simulink model "REGISTROS_64_BITS_02"  (R2022a)
settings: Solver=VariableStepAuto  StartTime=0.0  StopTime=10.0  RelTol=1e-3
undefined symbols (not defined in the file or in its folder): xc7z010iclg225
libraries: hdlBasic x6609, vmcUtilities x1
(part 20 of 23)

== system REGISTROS_64_BITS_02/REGISTRO_64_BITS_2/Q_OUT_32_BIT1 ==
  Q_OUT_0 (1 BIT) : Inport
  Q_OUT_1 (1 BIT) : Inport  Port=2
  Q_OUT_2 (1 BIT) : Inport  Port=3
  Q_OUT_3 (1 BIT) : Inport  Port=4
  Q_OUT_4 (1 BIT) : Inport  Port=5
  Q_OUT_5 (1 BIT) : Inport  Port=6
  Q_OUT_6 (1 BIT) : Inport  Port=7
  Q_OUT_7 (1 BIT) : Inport  Port=8
  Q_OUT_8 (1 BIT) : Inport  Port=9
  Q_OUT_9 (1 BIT) : Inport  Port=10
  Q_OUT_10 (1 BIT) : Inport  Port=11
  Q_OUT_11 (1 BIT) : Inport  Port=12
  Q_OUT_12 (1 BIT) : Inport  Port=13
  Q_OUT_13 (1 BIT) : Inport  Port=14
  Q_OUT_14 (1 BIT) : Inport  Port=15
  Q_OUT_15 (1 BIT) : Inport  Port=16
  Q_OUT_16 (1 BIT) : Inport  Port=17
  Q_OUT_17 (1 BIT) : Inport  Port=18
  Q_OUT_18 (1 BIT) : Inport  Port=19
  Q_OUT_19 (1 BIT) : Inport  Port=20
  Q_OUT_20 (1 BIT) : Inport  Port=21
  Q_OUT_21 (1 BIT) : Inport  Port=22
  Q_OUT_22 (1 BIT) : Inport  Port=23
  Q_OUT_23 (1 BIT) : Inport  Port=24
  Q_OUT_24 (1 BIT) : Inport  Port=25
  Q_OUT_25 (1 BIT) : Inport  Port=26
  Q_OUT_26 (1 BIT) : Inport  Port=27
  Q_OUT_27 (1 BIT) : Inport  Port=28
  Q_OUT_28 (1 BIT) : Inport  Port=29
  Q_OUT_29 (1 BIT) : Inport  Port=30
  Q_OUT_30 (1 BIT) : Inport  Port=31
  Q_OUT_31 (1 BIT) : Inport  Port=32
  Concat{1,3,6,8..30} (26 alike) : hdlBasic/Concat  num_inputs=2  XmcBlockStatus=1  maskContainerNames=group1  block_type=concat  block_config=sysgen:Concat_config
  IN_00 : hdlBasic/Concat  num_inputs=2  XmcBlockStatus=1  maskContainerNames=group1  block_type=concat  block_config=sysgen:Concat_config
  IN_01 : hdlBasic/Concat  num_inputs=2  XmcBlockStatus=1  maskContainerNames=group1  block_type=concat  block_config=sysgen:Concat_config
  IN_02 : hdlBasic/Concat  num_inputs=2  XmcBlockStatus=1  maskContainerNames=group1  block_type=concat  block_config=sysgen:Concat_config
  IN_03 : hdlBasic/Concat  num_inputs=2  XmcBlockStatus=1  maskContainerNames=group1  block_type=concat  block_config=sysgen:Concat_config
  IN_04 : hdlBasic/Concat  num_inputs=2  XmcBlockStatus=1  maskContainerNames=group1  block_type=concat  block_config=sysgen:Concat_config
  Q (32 BIT) : Outport
  wires:
  IN_01/1 -> Concat3/2
  Concat10/1 -> Concat12/1
  Concat27/1 -> Concat20/2
  Concat19/1 -> Concat21/2
  Concat22/1 -> Concat1/2
  Concat28/1 -> Concat30/1
  Concat11/1 -> Concat12/2
  Concat29/1 -> Concat30/2
  Concat21/1 -> Concat22/2
  IN_00/1 -> Concat3/1
  Concat3/1 -> Concat13/1
  Concat20/1 -> Concat22/1
  Concat17/1 -> Concat19/1
  Concat26/1 -> Concat27/2
  Concat6/1 -> Concat13/2
  Concat13/1 -> Concat15/1
  Concat30/1 -> Concat21/1
  Concat24/1 -> Concat20/1
  Concat16/1 -> Concat24/1
  Concat23/1 -> Concat24/2
  Concat18/1 -> Concat19/2
  Concat25/1 -> Concat27/1
  IN_02/1 -> Concat6/1
  IN_03/1 -> Concat6/2
  Concat9/1 -> Concat14/1
  Concat15/1 -> Concat1/1
  Concat8/1 -> Concat9/2
  IN_04/1 -> Concat9/1
  Concat14/1 -> Concat15/2
  Concat12/1 -> Concat14/2
  Concat1/1 -> Q (32 BIT)/1
  Q_OUT_31 (1 BIT)/1 -> IN_00/1
  Q_OUT_30 (1 BIT)/1 -> IN_00/2
  Q_OUT_29 (1 BIT)/1 -> IN_01/1
  Q_OUT_28 (1 BIT)/1 -> IN_01/2
  Q_OUT_27 (1 BIT)/1 -> IN_02/1
  Q_OUT_26 (1 BIT)/1 -> IN_02/2
  Q_OUT_25 (1 BIT)/1 -> IN_03/1
  Q_OUT_24 (1 BIT)/1 -> IN_03/2
  Q_OUT_23 (1 BIT)/1 -> IN_04/1
  Q_OUT_22 (1 BIT)/1 -> IN_04/2
  Q_OUT_21 (1 BIT)/1 -> Concat8/1
  Q_OUT_20 (1 BIT)/1 -> Concat8/2
  Q_OUT_19 (1 BIT)/1 -> Concat10/1
  Q_OUT_18 (1 BIT)/1 -> Concat10/2
  Q_OUT_17 (1 BIT)/1 -> Concat11/1
  Q_OUT_16 (1 BIT)/1 -> Concat11/2
  Q_OUT_15 (1 BIT)/1 -> Concat16/1
  Q_OUT_14 (1 BIT)/1 -> Concat16/2
  Q_OUT_13 (1 BIT)/1 -> Concat23/1
  Q_OUT_12 (1 BIT)/1 -> Concat23/2
  Q_OUT_11 (1 BIT)/1 -> Concat25/1
  Q_OUT_10 (1 BIT)/1 -> Concat25/2
  Q_OUT_9 (1 BIT)/1 -> Concat26/1
  Q_OUT_8 (1 BIT)/1 -> Concat26/2
  Q_OUT_7 (1 BIT)/1 -> Concat28/1
  Q_OUT_6 (1 BIT)/1 -> Concat28/2
  Q_OUT_5 (1 BIT)/1 -> Concat29/1
  Q_OUT_4 (1 BIT)/1 -> Concat29/2
  Q_OUT_3 (1 BIT)/1 -> Concat17/1
  Q_OUT_2 (1 BIT)/1 -> Concat17/2
  Q_OUT_1 (1 BIT)/1 -> Concat18/1
  Q_OUT_0 (1 BIT)/1 -> Concat18/2

== system REGISTROS_64_BITS_02/REGISTRO_64_BITS_2/Q_OUT_32_BIT2 ==
  Q_OUT_0 (1 BIT) : Inport
  Q_OUT_1 (1 BIT) : Inport  Port=2
  Q_OUT_2 (1 BIT) : Inport  Port=3
  Q_OUT_3 (1 BIT) : Inport  Port=4
  Q_OUT_4 (1 BIT) : Inport  Port=5
  Q_OUT_5 (1 BIT) : Inport  Port=6
  Q_OUT_6 (1 BIT) : Inport  Port=7
  Q_OUT_7 (1 BIT) : Inport  Port=8
  Q_OUT_8 (1 BIT) : Inport  Port=9
  Q_OUT_9 (1 BIT) : Inport  Port=10
  Q_OUT_10 (1 BIT) : Inport  Port=11
  Q_OUT_11 (1 BIT) : Inport  Port=12
  Q_OUT_12 (1 BIT) : Inport  Port=13
  Q_OUT_13 (1 BIT) : Inport  Port=14
  Q_OUT_14 (1 BIT) : Inport  Port=15
  Q_OUT_15 (1 BIT) : Inport  Port=16
  Q_OUT_16 (1 BIT) : Inport  Port=17
  Q_OUT_17 (1 BIT) : Inport  Port=18
  Q_OUT_18 (1 BIT) : Inport  Port=19
  Q_OUT_19 (1 BIT) : Inport  Port=20
  Q_OUT_20 (1 BIT) : Inport  Port=21
  Q_OUT_21 (1 BIT) : Inport  Port=22
  Q_OUT_22 (1 BIT) : Inport  Port=23
  Q_OUT_23 (1 BIT) : Inport  Port=24
  Q_OUT_24 (1 BIT) : Inport  Port=25
  Q_OUT_25 (1 BIT) : Inport  Port=26
  Q_OUT_26 (1 BIT) : Inport  Port=27
  Q_OUT_27 (1 BIT) : Inport  Port=28
  Q_OUT_28 (1 BIT) : Inport  Port=29
  Q_OUT_29 (1 BIT) : Inport  Port=30
  Q_OUT_30 (1 BIT) : Inport  Port=31
  Q_OUT_31 (1 BIT) : Inport  Port=32
  Concat{1,3,6,8..30} (26 alike) : hdlBasic/Concat  num_inputs=2  XmcBlockStatus=1  maskContainerNames=group1  block_type=concat  block_config=sysgen:Concat_config
  IN_00 : hdlBasic/Concat  num_inputs=2  XmcBlockStatus=1  maskContainerNames=group1  block_type=concat  block_config=sysgen:Concat_config
  IN_01 : hdlBasic/Concat  num_inputs=2  XmcBlockStatus=1  maskContainerNames=group1  block_type=concat  block_config=sysgen:Concat_config
  IN_02 : hdlBasic/Concat  num_inputs=2  XmcBlockStatus=1  maskContainerNames=group1  block_type=concat  block_config=sysgen:Concat_config
  IN_03 : hdlBasic/Concat  num_inputs=2  XmcBlockStatus=1  maskContainerNames=group1  block_type=concat  block_config=sysgen:Concat_config
  IN_04 : hdlBasic/Concat  num_inputs=2  XmcBlockStatus=1  maskContainerNames=group1  block_type=concat  block_config=sysgen:Concat_config
  Q (32 BIT) : Outport
  wires:
  IN_01/1 -> Concat3/2
  Concat10/1 -> Concat12/1
  Concat27/1 -> Concat20/2
  Concat19/1 -> Concat21/2
  Concat22/1 -> Concat1/2
  Concat28/1 -> Concat30/1
  Concat11/1 -> Concat12/2
  Concat29/1 -> Concat30/2
  Concat21/1 -> Concat22/2
  IN_00/1 -> Concat3/1
  Concat3/1 -> Concat13/1
  Concat20/1 -> Concat22/1
  Concat17/1 -> Concat19/1
  Concat26/1 -> Concat27/2
  Concat6/1 -> Concat13/2
  Concat13/1 -> Concat15/1
  Concat30/1 -> Concat21/1
  Concat24/1 -> Concat20/1
  Concat16/1 -> Concat24/1
  Concat23/1 -> Concat24/2
  Concat18/1 -> Concat19/2
  Concat25/1 -> Concat27/1
  IN_02/1 -> Concat6/1
  IN_03/1 -> Concat6/2
  Concat9/1 -> Concat14/1
  Concat15/1 -> Concat1/1
  Concat8/1 -> Concat9/2
  IN_04/1 -> Concat9/1
  Concat14/1 -> Concat15/2
  Concat12/1 -> Concat14/2
  Concat1/1 -> Q (32 BIT)/1
  Q_OUT_31 (1 BIT)/1 -> IN_00/1
  Q_OUT_30 (1 BIT)/1 -> IN_00/2
  Q_OUT_29 (1 BIT)/1 -> IN_01/1
  Q_OUT_28 (1 BIT)/1 -> IN_01/2
  Q_OUT_27 (1 BIT)/1 -> IN_02/1
  Q_OUT_26 (1 BIT)/1 -> IN_02/2
  Q_OUT_25 (1 BIT)/1 -> IN_03/1
  Q_OUT_24 (1 BIT)/1 -> IN_03/2
  Q_OUT_23 (1 BIT)/1 -> IN_04/1
  Q_OUT_22 (1 BIT)/1 -> IN_04/2
  Q_OUT_21 (1 BIT)/1 -> Concat8/1
  Q_OUT_20 (1 BIT)/1 -> Concat8/2
  Q_OUT_19 (1 BIT)/1 -> Concat10/1
  Q_OUT_18 (1 BIT)/1 -> Concat10/2
  Q_OUT_17 (1 BIT)/1 -> Concat11/1
  Q_OUT_16 (1 BIT)/1 -> Concat11/2
  Q_OUT_15 (1 BIT)/1 -> Concat16/1
  Q_OUT_14 (1 BIT)/1 -> Concat16/2
  Q_OUT_13 (1 BIT)/1 -> Concat23/1
  Q_OUT_12 (1 BIT)/1 -> Concat23/2
  Q_OUT_11 (1 BIT)/1 -> Concat25/1
  Q_OUT_10 (1 BIT)/1 -> Concat25/2
  Q_OUT_9 (1 BIT)/1 -> Concat26/1
  Q_OUT_8 (1 BIT)/1 -> Concat26/2
  Q_OUT_7 (1 BIT)/1 -> Concat28/1
  Q_OUT_6 (1 BIT)/1 -> Concat28/2
  Q_OUT_5 (1 BIT)/1 -> Concat29/1
  Q_OUT_4 (1 BIT)/1 -> Concat29/2
  Q_OUT_3 (1 BIT)/1 -> Concat17/1
  Q_OUT_2 (1 BIT)/1 -> Concat17/2
  Q_OUT_1 (1 BIT)/1 -> Concat18/1
  Q_OUT_0 (1 BIT)/1 -> Concat18/2

== system REGISTROS_64_BITS_02/REGISTRO_64_BITS_20/Q_OUT_32_BIT1 ==
  Q_OUT_0 (1 BIT) : Inport
  Q_OUT_1 (1 BIT) : Inport  Port=2
  Q_OUT_2 (1 BIT) : Inport  Port=3
  Q_OUT_3 (1 BIT) : Inport  Port=4
  Q_OUT_4 (1 BIT) : Inport  Port=5
  Q_OUT_5 (1 BIT) : Inport  Port=6
  Q_OUT_6 (1 BIT) : Inport  Port=7
  Q_OUT_7 (1 BIT) : Inport  Port=8
  Q_OUT_8 (1 BIT) : Inport  Port=9
  Q_OUT_9 (1 BIT) : Inport  Port=10
  Q_OUT_10 (1 BIT) : Inport  Port=11
  Q_OUT_11 (1 BIT) : Inport  Port=12
  Q_OUT_12 (1 BIT) : Inport  Port=13
  Q_OUT_13 (1 BIT) : Inport  Port=14
  Q_OUT_14 (1 BIT) : Inport  Port=15
  Q_OUT_15 (1 BIT) : Inport  Port=16
  Q_OUT_16 (1 BIT) : Inport  Port=17
  Q_OUT_17 (1 BIT) : Inport  Port=18
  Q_OUT_18 (1 BIT) : Inport  Port=19
  Q_OUT_19 (1 BIT) : Inport  Port=20
  Q_OUT_20 (1 BIT) : Inport  Port=21
  Q_OUT_21 (1 BIT) : Inport  Port=22
  Q_OUT_22 (1 BIT) : Inport  Port=23
  Q_OUT_23 (1 BIT) : Inport  Port=24
  Q_OUT_24 (1 BIT) : Inport  Port=25
  Q_OUT_25 (1 BIT) : Inport  Port=26
  Q_OUT_26 (1 BIT) : Inport  Port=27
  Q_OUT_27 (1 BIT) : Inport  Port=28
  Q_OUT_28 (1 BIT) : Inport  Port=29
  Q_OUT_29 (1 BIT) : Inport  Port=30
  Q_OUT_30 (1 BIT) : Inport  Port=31
  Q_OUT_31 (1 BIT) : Inport  Port=32
  Concat{1,3,6,8..30} (26 alike) : hdlBasic/Concat  num_inputs=2  XmcBlockStatus=1  maskContainerNames=group1  block_type=concat  block_config=sysgen:Concat_config
  IN_00 : hdlBasic/Concat  num_inputs=2  XmcBlockStatus=1  maskContainerNames=group1  block_type=concat  block_config=sysgen:Concat_config
  IN_01 : hdlBasic/Concat  num_inputs=2  XmcBlockStatus=1  maskContainerNames=group1  block_type=concat  block_config=sysgen:Concat_config
  IN_02 : hdlBasic/Concat  num_inputs=2  XmcBlockStatus=1  maskContainerNames=group1  block_type=concat  block_config=sysgen:Concat_config
  IN_03 : hdlBasic/Concat  num_inputs=2  XmcBlockStatus=1  maskContainerNames=group1  block_type=concat  block_config=sysgen:Concat_config
  IN_04 : hdlBasic/Concat  num_inputs=2  XmcBlockStatus=1  maskContainerNames=group1  block_type=concat  block_config=sysgen:Concat_config
  Q (32 BIT) : Outport
  wires:
  IN_01/1 -> Concat3/2
  Concat10/1 -> Concat12/1
  Concat27/1 -> Concat20/2
  Concat19/1 -> Concat21/2
  Concat22/1 -> Concat1/2
  Concat28/1 -> Concat30/1
  Concat11/1 -> Concat12/2
  Concat29/1 -> Concat30/2
  Concat21/1 -> Concat22/2
  IN_00/1 -> Concat3/1
  Concat3/1 -> Concat13/1
  Concat20/1 -> Concat22/1
  Concat17/1 -> Concat19/1
  Concat26/1 -> Concat27/2
  Concat6/1 -> Concat13/2
  Concat13/1 -> Concat15/1
  Concat30/1 -> Concat21/1
  Concat24/1 -> Concat20/1
  Concat16/1 -> Concat24/1
  Concat23/1 -> Concat24/2
  Concat18/1 -> Concat19/2
  Concat25/1 -> Concat27/1
  IN_02/1 -> Concat6/1
  IN_03/1 -> Concat6/2
  Concat9/1 -> Concat14/1
  Concat15/1 -> Concat1/1
  Concat8/1 -> Concat9/2
  IN_04/1 -> Concat9/1
  Concat14/1 -> Concat15/2
  Concat12/1 -> Concat14/2
  Concat1/1 -> Q (32 BIT)/1
  Q_OUT_31 (1 BIT)/1 -> IN_00/1
  Q_OUT_30 (1 BIT)/1 -> IN_00/2
  Q_OUT_29 (1 BIT)/1 -> IN_01/1
  Q_OUT_28 (1 BIT)/1 -> IN_01/2
  Q_OUT_27 (1 BIT)/1 -> IN_02/1
  Q_OUT_26 (1 BIT)/1 -> IN_02/2
  Q_OUT_25 (1 BIT)/1 -> IN_03/1
  Q_OUT_24 (1 BIT)/1 -> IN_03/2
  Q_OUT_23 (1 BIT)/1 -> IN_04/1
  Q_OUT_22 (1 BIT)/1 -> IN_04/2
  Q_OUT_21 (1 BIT)/1 -> Concat8/1
  Q_OUT_20 (1 BIT)/1 -> Concat8/2
  Q_OUT_19 (1 BIT)/1 -> Concat10/1
  Q_OUT_18 (1 BIT)/1 -> Concat10/2
  Q_OUT_17 (1 BIT)/1 -> Concat11/1
  Q_OUT_16 (1 BIT)/1 -> Concat11/2
  Q_OUT_15 (1 BIT)/1 -> Concat16/1
  Q_OUT_14 (1 BIT)/1 -> Concat16/2
  Q_OUT_13 (1 BIT)/1 -> Concat23/1
  Q_OUT_12 (1 BIT)/1 -> Concat23/2
  Q_OUT_11 (1 BIT)/1 -> Concat25/1
  Q_OUT_10 (1 BIT)/1 -> Concat25/2
  Q_OUT_9 (1 BIT)/1 -> Concat26/1
  Q_OUT_8 (1 BIT)/1 -> Concat26/2
  Q_OUT_7 (1 BIT)/1 -> Concat28/1
  Q_OUT_6 (1 BIT)/1 -> Concat28/2
  Q_OUT_5 (1 BIT)/1 -> Concat29/1
  Q_OUT_4 (1 BIT)/1 -> Concat29/2
  Q_OUT_3 (1 BIT)/1 -> Concat17/1
  Q_OUT_2 (1 BIT)/1 -> Concat17/2
  Q_OUT_1 (1 BIT)/1 -> Concat18/1
  Q_OUT_0 (1 BIT)/1 -> Concat18/2

== system REGISTROS_64_BITS_02/REGISTRO_64_BITS_20/Q_OUT_32_BIT2 ==
  Q_OUT_0 (1 BIT) : Inport
  Q_OUT_1 (1 BIT) : Inport  Port=2
  Q_OUT_2 (1 BIT) : Inport  Port=3
  Q_OUT_3 (1 BIT) : Inport  Port=4
  Q_OUT_4 (1 BIT) : Inport  Port=5
  Q_OUT_5 (1 BIT) : Inport  Port=6
  Q_OUT_6 (1 BIT) : Inport  Port=7
  Q_OUT_7 (1 BIT) : Inport  Port=8
  Q_OUT_8 (1 BIT) : Inport  Port=9
  Q_OUT_9 (1 BIT) : Inport  Port=10
  Q_OUT_10 (1 BIT) : Inport  Port=11
  Q_OUT_11 (1 BIT) : Inport  Port=12
  Q_OUT_12 (1 BIT) : Inport  Port=13
  Q_OUT_13 (1 BIT) : Inport  Port=14
  Q_OUT_14 (1 BIT) : Inport  Port=15
  Q_OUT_15 (1 BIT) : Inport  Port=16
  Q_OUT_16 (1 BIT) : Inport  Port=17
  Q_OUT_17 (1 BIT) : Inport  Port=18
  Q_OUT_18 (1 BIT) : Inport  Port=19
  Q_OUT_19 (1 BIT) : Inport  Port=20
  Q_OUT_20 (1 BIT) : Inport  Port=21
  Q_OUT_21 (1 BIT) : Inport  Port=22
  Q_OUT_22 (1 BIT) : Inport  Port=23
  Q_OUT_23 (1 BIT) : Inport  Port=24
  Q_OUT_24 (1 BIT) : Inport  Port=25
  Q_OUT_25 (1 BIT) : Inport  Port=26
  Q_OUT_26 (1 BIT) : Inport  Port=27
  Q_OUT_27 (1 BIT) : Inport  Port=28
  Q_OUT_28 (1 BIT) : Inport  Port=29
  Q_OUT_29 (1 BIT) : Inport  Port=30
  Q_OUT_30 (1 BIT) : Inport  Port=31
  Q_OUT_31 (1 BIT) : Inport  Port=32
  Concat{1,3,6,8..30} (26 alike) : hdlBasic/Concat  num_inputs=2  XmcBlockStatus=1  maskContainerNames=group1  block_type=concat  block_config=sysgen:Concat_config
  IN_00 : hdlBasic/Concat  num_inputs=2  XmcBlockStatus=1  maskContainerNames=group1  block_type=concat  block_config=sysgen:Concat_config
  IN_01 : hdlBasic/Concat  num_inputs=2  XmcBlockStatus=1  maskContainerNames=group1  block_type=concat  block_config=sysgen:Concat_config
  IN_02 : hdlBasic/Concat  num_inputs=2  XmcBlockStatus=1  maskContainerNames=group1  block_type=concat  block_config=sysgen:Concat_config
  IN_03 : hdlBasic/Concat  num_inputs=2  XmcBlockStatus=1  maskContainerNames=group1  block_type=concat  block_config=sysgen:Concat_config
  IN_04 : hdlBasic/Concat  num_inputs=2  XmcBlockStatus=1  maskContainerNames=group1  block_type=concat  block_config=sysgen:Concat_config
  Q (32 BIT) : Outport
  wires:
  IN_01/1 -> Concat3/2
  Concat10/1 -> Concat12/1
  Concat27/1 -> Concat20/2
  Concat19/1 -> Concat21/2
  Concat22/1 -> Concat1/2
  Concat28/1 -> Concat30/1
  Concat11/1 -> Concat12/2
  Concat29/1 -> Concat30/2
  Concat21/1 -> Concat22/2
  IN_00/1 -> Concat3/1
  Concat3/1 -> Concat13/1
  Concat20/1 -> Concat22/1
  Concat17/1 -> Concat19/1
  Concat26/1 -> Concat27/2
  Concat6/1 -> Concat13/2
  Concat13/1 -> Concat15/1
  Concat30/1 -> Concat21/1
  Concat24/1 -> Concat20/1
  Concat16/1 -> Concat24/1
  Concat23/1 -> Concat24/2
  Concat18/1 -> Concat19/2
  Concat25/1 -> Concat27/1
  IN_02/1 -> Concat6/1
  IN_03/1 -> Concat6/2
  Concat9/1 -> Concat14/1
  Concat15/1 -> Concat1/1
  Concat8/1 -> Concat9/2
  IN_04/1 -> Concat9/1
  Concat14/1 -> Concat15/2
  Concat12/1 -> Concat14/2
  Concat1/1 -> Q (32 BIT)/1
  Q_OUT_31 (1 BIT)/1 -> IN_00/1
  Q_OUT_30 (1 BIT)/1 -> IN_00/2
  Q_OUT_29 (1 BIT)/1 -> IN_01/1
  Q_OUT_28 (1 BIT)/1 -> IN_01/2
  Q_OUT_27 (1 BIT)/1 -> IN_02/1
  Q_OUT_26 (1 BIT)/1 -> IN_02/2
  Q_OUT_25 (1 BIT)/1 -> IN_03/1
  Q_OUT_24 (1 BIT)/1 -> IN_03/2
  Q_OUT_23 (1 BIT)/1 -> IN_04/1
  Q_OUT_22 (1 BIT)/1 -> IN_04/2
  Q_OUT_21 (1 BIT)/1 -> Concat8/1
  Q_OUT_20 (1 BIT)/1 -> Concat8/2
  Q_OUT_19 (1 BIT)/1 -> Concat10/1
  Q_OUT_18 (1 BIT)/1 -> Concat10/2
  Q_OUT_17 (1 BIT)/1 -> Concat11/1
  Q_OUT_16 (1 BIT)/1 -> Concat11/2
  Q_OUT_15 (1 BIT)/1 -> Concat16/1
  Q_OUT_14 (1 BIT)/1 -> Concat16/2
  Q_OUT_13 (1 BIT)/1 -> Concat23/1
  Q_OUT_12 (1 BIT)/1 -> Concat23/2
  Q_OUT_11 (1 BIT)/1 -> Concat25/1
  Q_OUT_10 (1 BIT)/1 -> Concat25/2
  Q_OUT_9 (1 BIT)/1 -> Concat26/1
  Q_OUT_8 (1 BIT)/1 -> Concat26/2
  Q_OUT_7 (1 BIT)/1 -> Concat28/1
  Q_OUT_6 (1 BIT)/1 -> Concat28/2
  Q_OUT_5 (1 BIT)/1 -> Concat29/1
  Q_OUT_4 (1 BIT)/1 -> Concat29/2
  Q_OUT_3 (1 BIT)/1 -> Concat17/1
  Q_OUT_2 (1 BIT)/1 -> Concat17/2
  Q_OUT_1 (1 BIT)/1 -> Concat18/1
  Q_OUT_0 (1 BIT)/1 -> Concat18/2

== system REGISTROS_64_BITS_02/REGISTRO_64_BITS_21/Q_OUT_32_BIT1 ==
  Q_OUT_0 (1 BIT) : Inport
  Q_OUT_1 (1 BIT) : Inport  Port=2
  Q_OUT_2 (1 BIT) : Inport  Port=3
  Q_OUT_3 (1 BIT) : Inport  Port=4
  Q_OUT_4 (1 BIT) : Inport  Port=5
  Q_OUT_5 (1 BIT) : Inport  Port=6
  Q_OUT_6 (1 BIT) : Inport  Port=7
  Q_OUT_7 (1 BIT) : Inport  Port=8
  Q_OUT_8 (1 BIT) : Inport  Port=9
  Q_OUT_9 (1 BIT) : Inport  Port=10
  Q_OUT_10 (1 BIT) : Inport  Port=11
  Q_OUT_11 (1 BIT) : Inport  Port=12
  Q_OUT_12 (1 BIT) : Inport  Port=13
  Q_OUT_13 (1 BIT) : Inport  Port=14
  Q_OUT_14 (1 BIT) : Inport  Port=15
  Q_OUT_15 (1 BIT) : Inport  Port=16
  Q_OUT_16 (1 BIT) : Inport  Port=17
  Q_OUT_17 (1 BIT) : Inport  Port=18
  Q_OUT_18 (1 BIT) : Inport  Port=19
  Q_OUT_19 (1 BIT) : Inport  Port=20
  Q_OUT_20 (1 BIT) : Inport  Port=21
  Q_OUT_21 (1 BIT) : Inport  Port=22
  Q_OUT_22 (1 BIT) : Inport  Port=23
  Q_OUT_23 (1 BIT) : Inport  Port=24
  Q_OUT_24 (1 BIT) : Inport  Port=25
  Q_OUT_25 (1 BIT) : Inport  Port=26
  Q_OUT_26 (1 BIT) : Inport  Port=27
  Q_OUT_27 (1 BIT) : Inport  Port=28
  Q_OUT_28 (1 BIT) : Inport  Port=29
  Q_OUT_29 (1 BIT) : Inport  Port=30
  Q_OUT_30 (1 BIT) : Inport  Port=31
  Q_OUT_31 (1 BIT) : Inport  Port=32
  Concat{1,3,6,8..30} (26 alike) : hdlBasic/Concat  num_inputs=2  XmcBlockStatus=1  maskContainerNames=group1  block_type=concat  block_config=sysgen:Concat_config
  IN_00 : hdlBasic/Concat  num_inputs=2  XmcBlockStatus=1  maskContainerNames=group1  block_type=concat  block_config=sysgen:Concat_config
  IN_01 : hdlBasic/Concat  num_inputs=2  XmcBlockStatus=1  maskContainerNames=group1  block_type=concat  block_config=sysgen:Concat_config
  IN_02 : hdlBasic/Concat  num_inputs=2  XmcBlockStatus=1  maskContainerNames=group1  block_type=concat  block_config=sysgen:Concat_config
  IN_03 : hdlBasic/Concat  num_inputs=2  XmcBlockStatus=1  maskContainerNames=group1  block_type=concat  block_config=sysgen:Concat_config
  IN_04 : hdlBasic/Concat  num_inputs=2  XmcBlockStatus=1  maskContainerNames=group1  block_type=concat  block_config=sysgen:Concat_config
  Q (32 BIT) : Outport
  wires:
  IN_01/1 -> Concat3/2
  Concat10/1 -> Concat12/1
  Concat27/1 -> Concat20/2
  Concat19/1 -> Concat21/2
  Concat22/1 -> Concat1/2
  Concat28/1 -> Concat30/1
  Concat11/1 -> Concat12/2
  Concat29/1 -> Concat30/2
  Concat21/1 -> Concat22/2
  IN_00/1 -> Concat3/1
  Concat3/1 -> Concat13/1
  Concat20/1 -> Concat22/1
  Concat17/1 -> Concat19/1
  Concat26/1 -> Concat27/2
  Concat6/1 -> Concat13/2
  Concat13/1 -> Concat15/1
  Concat30/1 -> Concat21/1
  Concat24/1 -> Concat20/1
  Concat16/1 -> Concat24/1
  Concat23/1 -> Concat24/2
  Concat18/1 -> Concat19/2
  Concat25/1 -> Concat27/1
  IN_02/1 -> Concat6/1
  IN_03/1 -> Concat6/2
  Concat9/1 -> Concat14/1
  Concat15/1 -> Concat1/1
  Concat8/1 -> Concat9/2
  IN_04/1 -> Concat9/1
  Concat14/1 -> Concat15/2
  Concat12/1 -> Concat14/2
  Concat1/1 -> Q (32 BIT)/1
  Q_OUT_31 (1 BIT)/1 -> IN_00/1
  Q_OUT_30 (1 BIT)/1 -> IN_00/2
  Q_OUT_29 (1 BIT)/1 -> IN_01/1
  Q_OUT_28 (1 BIT)/1 -> IN_01/2
  Q_OUT_27 (1 BIT)/1 -> IN_02/1
  Q_OUT_26 (1 BIT)/1 -> IN_02/2
  Q_OUT_25 (1 BIT)/1 -> IN_03/1
  Q_OUT_24 (1 BIT)/1 -> IN_03/2
  Q_OUT_23 (1 BIT)/1 -> IN_04/1
  Q_OUT_22 (1 BIT)/1 -> IN_04/2
  Q_OUT_21 (1 BIT)/1 -> Concat8/1
  Q_OUT_20 (1 BIT)/1 -> Concat8/2
  Q_OUT_19 (1 BIT)/1 -> Concat10/1
  Q_OUT_18 (1 BIT)/1 -> Concat10/2
  Q_OUT_17 (1 BIT)/1 -> Concat11/1
  Q_OUT_16 (1 BIT)/1 -> Concat11/2
  Q_OUT_15 (1 BIT)/1 -> Concat16/1
  Q_OUT_14 (1 BIT)/1 -> Concat16/2
  Q_OUT_13 (1 BIT)/1 -> Concat23/1
  Q_OUT_12 (1 BIT)/1 -> Concat23/2
  Q_OUT_11 (1 BIT)/1 -> Concat25/1
  Q_OUT_10 (1 BIT)/1 -> Concat25/2
  Q_OUT_9 (1 BIT)/1 -> Concat26/1
  Q_OUT_8 (1 BIT)/1 -> Concat26/2
  Q_OUT_7 (1 BIT)/1 -> Concat28/1
  Q_OUT_6 (1 BIT)/1 -> Concat28/2
  Q_OUT_5 (1 BIT)/1 -> Concat29/1
  Q_OUT_4 (1 BIT)/1 -> Concat29/2
  Q_OUT_3 (1 BIT)/1 -> Concat17/1
  Q_OUT_2 (1 BIT)/1 -> Concat17/2
  Q_OUT_1 (1 BIT)/1 -> Concat18/1
  Q_OUT_0 (1 BIT)/1 -> Concat18/2

== system REGISTROS_64_BITS_02/REGISTRO_64_BITS_21/Q_OUT_32_BIT2 ==
  Q_OUT_0 (1 BIT) : Inport
  Q_OUT_1 (1 BIT) : Inport  Port=2
  Q_OUT_2 (1 BIT) : Inport  Port=3
  Q_OUT_3 (1 BIT) : Inport  Port=4
  Q_OUT_4 (1 BIT) : Inport  Port=5
  Q_OUT_5 (1 BIT) : Inport  Port=6
  Q_OUT_6 (1 BIT) : Inport  Port=7
  Q_OUT_7 (1 BIT) : Inport  Port=8
  Q_OUT_8 (1 BIT) : Inport  Port=9
  Q_OUT_9 (1 BIT) : Inport  Port=10
  Q_OUT_10 (1 BIT) : Inport  Port=11
  Q_OUT_11 (1 BIT) : Inport  Port=12
  Q_OUT_12 (1 BIT) : Inport  Port=13
  Q_OUT_13 (1 BIT) : Inport  Port=14
  Q_OUT_14 (1 BIT) : Inport  Port=15
  Q_OUT_15 (1 BIT) : Inport  Port=16
  Q_OUT_16 (1 BIT) : Inport  Port=17
  Q_OUT_17 (1 BIT) : Inport  Port=18
  Q_OUT_18 (1 BIT) : Inport  Port=19
  Q_OUT_19 (1 BIT) : Inport  Port=20
  Q_OUT_20 (1 BIT) : Inport  Port=21
  Q_OUT_21 (1 BIT) : Inport  Port=22
  Q_OUT_22 (1 BIT) : Inport  Port=23
  Q_OUT_23 (1 BIT) : Inport  Port=24
  Q_OUT_24 (1 BIT) : Inport  Port=25
  Q_OUT_25 (1 BIT) : Inport  Port=26
  Q_OUT_26 (1 BIT) : Inport  Port=27
  Q_OUT_27 (1 BIT) : Inport  Port=28
  Q_OUT_28 (1 BIT) : Inport  Port=29
  Q_OUT_29 (1 BIT) : Inport  Port=30
  Q_OUT_30 (1 BIT) : Inport  Port=31
  Q_OUT_31 (1 BIT) : Inport  Port=32
  Concat{1,3,6,8..30} (26 alike) : hdlBasic/Concat  num_inputs=2  XmcBlockStatus=1  maskContainerNames=group1  block_type=concat  block_config=sysgen:Concat_config
  IN_00 : hdlBasic/Concat  num_inputs=2  XmcBlockStatus=1  maskContainerNames=group1  block_type=concat  block_config=sysgen:Concat_config
  IN_01 : hdlBasic/Concat  num_inputs=2  XmcBlockStatus=1  maskContainerNames=group1  block_type=concat  block_config=sysgen:Concat_config
  IN_02 : hdlBasic/Concat  num_inputs=2  XmcBlockStatus=1  maskContainerNames=group1  block_type=concat  block_config=sysgen:Concat_config
  IN_03 : hdlBasic/Concat  num_inputs=2  XmcBlockStatus=1  maskContainerNames=group1  block_type=concat  block_config=sysgen:Concat_config
  IN_04 : hdlBasic/Concat  num_inputs=2  XmcBlockStatus=1  maskContainerNames=group1  block_type=concat  block_config=sysgen:Concat_config
  Q (32 BIT) : Outport
  wires:
  IN_01/1 -> Concat3/2
  Concat10/1 -> Concat12/1
  Concat27/1 -> Concat20/2
  Concat19/1 -> Concat21/2
  Concat22/1 -> Concat1/2
  Concat28/1 -> Concat30/1
  Concat11/1 -> Concat12/2
  Concat29/1 -> Concat30/2
  Concat21/1 -> Concat22/2
  IN_00/1 -> Concat3/1
  Concat3/1 -> Concat13/1
  Concat20/1 -> Concat22/1
  Concat17/1 -> Concat19/1
  Concat26/1 -> Concat27/2
  Concat6/1 -> Concat13/2
  Concat13/1 -> Concat15/1
  Concat30/1 -> Concat21/1
  Concat24/1 -> Concat20/1
  Concat16/1 -> Concat24/1
  Concat23/1 -> Concat24/2
  Concat18/1 -> Concat19/2
  Concat25/1 -> Concat27/1
  IN_02/1 -> Concat6/1
  IN_03/1 -> Concat6/2
  Concat9/1 -> Concat14/1
  Concat15/1 -> Concat1/1
  Concat8/1 -> Concat9/2
  IN_04/1 -> Concat9/1
  Concat14/1 -> Concat15/2
  Concat12/1 -> Concat14/2
  Concat1/1 -> Q (32 BIT)/1
  Q_OUT_31 (1 BIT)/1 -> IN_00/1
  Q_OUT_30 (1 BIT)/1 -> IN_00/2
  Q_OUT_29 (1 BIT)/1 -> IN_01/1
  Q_OUT_28 (1 BIT)/1 -> IN_01/2
  Q_OUT_27 (1 BIT)/1 -> IN_02/1
  Q_OUT_26 (1 BIT)/1 -> IN_02/2
  Q_OUT_25 (1 BIT)/1 -> IN_03/1
  Q_OUT_24 (1 BIT)/1 -> IN_03/2
  Q_OUT_23 (1 BIT)/1 -> IN_04/1
  Q_OUT_22 (1 BIT)/1 -> IN_04/2
  Q_OUT_21 (1 BIT)/1 -> Concat8/1
  Q_OUT_20 (1 BIT)/1 -> Concat8/2
  Q_OUT_19 (1 BIT)/1 -> Concat10/1
  Q_OUT_18 (1 BIT)/1 -> Concat10/2
  Q_OUT_17 (1 BIT)/1 -> Concat11/1
  Q_OUT_16 (1 BIT)/1 -> Concat11/2
  Q_OUT_15 (1 BIT)/1 -> Concat16/1
  Q_OUT_14 (1 BIT)/1 -> Concat16/2
  Q_OUT_13 (1 BIT)/1 -> Concat23/1
  Q_OUT_12 (1 BIT)/1 -> Concat23/2
  Q_OUT_11 (1 BIT)/1 -> Concat25/1
  Q_OUT_10 (1 BIT)/1 -> Concat25/2
  Q_OUT_9 (1 BIT)/1 -> Concat26/1
  Q_OUT_8 (1 BIT)/1 -> Concat26/2
  Q_OUT_7 (1 BIT)/1 -> Concat28/1
  Q_OUT_6 (1 BIT)/1 -> Concat28/2
  Q_OUT_5 (1 BIT)/1 -> Concat29/1
  Q_OUT_4 (1 BIT)/1 -> Concat29/2
  Q_OUT_3 (1 BIT)/1 -> Concat17/1
  Q_OUT_2 (1 BIT)/1 -> Concat17/2
  Q_OUT_1 (1 BIT)/1 -> Concat18/1
  Q_OUT_0 (1 BIT)/1 -> Concat18/2

== system REGISTROS_64_BITS_02/REGISTRO_64_BITS_22/Q_OUT_32_BIT1 ==
  Q_OUT_0 (1 BIT) : Inport
  Q_OUT_1 (1 BIT) : Inport  Port=2
  Q_OUT_2 (1 BIT) : Inport  Port=3
  Q_OUT_3 (1 BIT) : Inport  Port=4
  Q_OUT_4 (1 BIT) : Inport  Port=5
  Q_OUT_5 (1 BIT) : Inport  Port=6
  Q_OUT_6 (1 BIT) : Inport  Port=7
  Q_OUT_7 (1 BIT) : Inport  Port=8
  Q_OUT_8 (1 BIT) : Inport  Port=9
  Q_OUT_9 (1 BIT) : Inport  Port=10
  Q_OUT_10 (1 BIT) : Inport  Port=11
  Q_OUT_11 (1 BIT) : Inport  Port=12
  Q_OUT_12 (1 BIT) : Inport  Port=13
  Q_OUT_13 (1 BIT) : Inport  Port=14
  Q_OUT_14 (1 BIT) : Inport  Port=15
  Q_OUT_15 (1 BIT) : Inport  Port=16
  Q_OUT_16 (1 BIT) : Inport  Port=17
  Q_OUT_17 (1 BIT) : Inport  Port=18
  Q_OUT_18 (1 BIT) : Inport  Port=19
  Q_OUT_19 (1 BIT) : Inport  Port=20
  Q_OUT_20 (1 BIT) : Inport  Port=21
  Q_OUT_21 (1 BIT) : Inport  Port=22
  Q_OUT_22 (1 BIT) : Inport  Port=23
  Q_OUT_23 (1 BIT) : Inport  Port=24
  Q_OUT_24 (1 BIT) : Inport  Port=25
  Q_OUT_25 (1 BIT) : Inport  Port=26
  Q_OUT_26 (1 BIT) : Inport  Port=27
  Q_OUT_27 (1 BIT) : Inport  Port=28
  Q_OUT_28 (1 BIT) : Inport  Port=29
  Q_OUT_29 (1 BIT) : Inport  Port=30
  Q_OUT_30 (1 BIT) : Inport  Port=31
  Q_OUT_31 (1 BIT) : Inport  Port=32
  Concat{1,3,6,8..30} (26 alike) : hdlBasic/Concat  num_inputs=2  XmcBlockStatus=1  maskContainerNames=group1  block_type=concat  block_config=sysgen:Concat_config
  IN_00 : hdlBasic/Concat  num_inputs=2  XmcBlockStatus=1  maskContainerNames=group1  block_type=concat  block_config=sysgen:Concat_config
  IN_01 : hdlBasic/Concat  num_inputs=2  XmcBlockStatus=1  maskContainerNames=group1  block_type=concat  block_config=sysgen:Concat_config
  IN_02 : hdlBasic/Concat  num_inputs=2  XmcBlockStatus=1  maskContainerNames=group1  block_type=concat  block_config=sysgen:Concat_config
  IN_03 : hdlBasic/Concat  num_inputs=2  XmcBlockStatus=1  maskContainerNames=group1  block_type=concat  block_config=sysgen:Concat_config
  IN_04 : hdlBasic/Concat  num_inputs=2  XmcBlockStatus=1  maskContainerNames=group1  block_type=concat  block_config=sysgen:Concat_config
  Q (32 BIT) : Outport
  wires:
  IN_01/1 -> Concat3/2
  Concat10/1 -> Concat12/1
  Concat27/1 -> Concat20/2
  Concat19/1 -> Concat21/2
  Concat22/1 -> Concat1/2
  Concat28/1 -> Concat30/1
  Concat11/1 -> Concat12/2
  Concat29/1 -> Concat30/2
  Concat21/1 -> Concat22/2
  IN_00/1 -> Concat3/1
  Concat3/1 -> Concat13/1
  Concat20/1 -> Concat22/1
  Concat17/1 -> Concat19/1
  Concat26/1 -> Concat27/2
  Concat6/1 -> Concat13/2
  Concat13/1 -> Concat15/1
  Concat30/1 -> Concat21/1
  Concat24/1 -> Concat20/1
  Concat16/1 -> Concat24/1
  Concat23/1 -> Concat24/2
  Concat18/1 -> Concat19/2
  Concat25/1 -> Concat27/1
  IN_02/1 -> Concat6/1
  IN_03/1 -> Concat6/2
  Concat9/1 -> Concat14/1
  Concat15/1 -> Concat1/1
  Concat8/1 -> Concat9/2
  IN_04/1 -> Concat9/1
  Concat14/1 -> Concat15/2
  Concat12/1 -> Concat14/2
  Concat1/1 -> Q (32 BIT)/1
  Q_OUT_31 (1 BIT)/1 -> IN_00/1
  Q_OUT_30 (1 BIT)/1 -> IN_00/2
  Q_OUT_29 (1 BIT)/1 -> IN_01/1
  Q_OUT_28 (1 BIT)/1 -> IN_01/2
  Q_OUT_27 (1 BIT)/1 -> IN_02/1
  Q_OUT_26 (1 BIT)/1 -> IN_02/2
  Q_OUT_25 (1 BIT)/1 -> IN_03/1
  Q_OUT_24 (1 BIT)/1 -> IN_03/2
  Q_OUT_23 (1 BIT)/1 -> IN_04/1
  Q_OUT_22 (1 BIT)/1 -> IN_04/2
  Q_OUT_21 (1 BIT)/1 -> Concat8/1
  Q_OUT_20 (1 BIT)/1 -> Concat8/2
  Q_OUT_19 (1 BIT)/1 -> Concat10/1
  Q_OUT_18 (1 BIT)/1 -> Concat10/2
  Q_OUT_17 (1 BIT)/1 -> Concat11/1
  Q_OUT_16 (1 BIT)/1 -> Concat11/2
  Q_OUT_15 (1 BIT)/1 -> Concat16/1
  Q_OUT_14 (1 BIT)/1 -> Concat16/2
  Q_OUT_13 (1 BIT)/1 -> Concat23/1
  Q_OUT_12 (1 BIT)/1 -> Concat23/2
  Q_OUT_11 (1 BIT)/1 -> Concat25/1
  Q_OUT_10 (1 BIT)/1 -> Concat25/2
  Q_OUT_9 (1 BIT)/1 -> Concat26/1
  Q_OUT_8 (1 BIT)/1 -> Concat26/2
  Q_OUT_7 (1 BIT)/1 -> Concat28/1
  Q_OUT_6 (1 BIT)/1 -> Concat28/2
  Q_OUT_5 (1 BIT)/1 -> Concat29/1
  Q_OUT_4 (1 BIT)/1 -> Concat29/2
  Q_OUT_3 (1 BIT)/1 -> Concat17/1
  Q_OUT_2 (1 BIT)/1 -> Concat17/2
  Q_OUT_1 (1 BIT)/1 -> Concat18/1
  Q_OUT_0 (1 BIT)/1 -> Concat18/2

== system REGISTROS_64_BITS_02/REGISTRO_64_BITS_22/Q_OUT_32_BIT2 ==
  Q_OUT_0 (1 BIT) : Inport
  Q_OUT_1 (1 BIT) : Inport  Port=2
  Q_OUT_2 (1 BIT) : Inport  Port=3
  Q_OUT_3 (1 BIT) : Inport  Port=4
  Q_OUT_4 (1 BIT) : Inport  Port=5
  Q_OUT_5 (1 BIT) : Inport  Port=6
  Q_OUT_6 (1 BIT) : Inport  Port=7
  Q_OUT_7 (1 BIT) : Inport  Port=8
  Q_OUT_8 (1 BIT) : Inport  Port=9
  Q_OUT_9 (1 BIT) : Inport  Port=10
  Q_OUT_10 (1 BIT) : Inport  Port=11
  Q_OUT_11 (1 BIT) : Inport  Port=12
  Q_OUT_12 (1 BIT) : Inport  Port=13
  Q_OUT_13 (1 BIT) : Inport  Port=14
  Q_OUT_14 (1 BIT) : Inport  Port=15
  Q_OUT_15 (1 BIT) : Inport  Port=16
  Q_OUT_16 (1 BIT) : Inport  Port=17
  Q_OUT_17 (1 BIT) : Inport  Port=18
  Q_OUT_18 (1 BIT) : Inport  Port=19
  Q_OUT_19 (1 BIT) : Inport  Port=20
  Q_OUT_20 (1 BIT) : Inport  Port=21
  Q_OUT_21 (1 BIT) : Inport  Port=22
  Q_OUT_22 (1 BIT) : Inport  Port=23
  Q_OUT_23 (1 BIT) : Inport  Port=24
  Q_OUT_24 (1 BIT) : Inport  Port=25
  Q_OUT_25 (1 BIT) : Inport  Port=26
  Q_OUT_26 (1 BIT) : Inport  Port=27
  Q_OUT_27 (1 BIT) : Inport  Port=28
  Q_OUT_28 (1 BIT) : Inport  Port=29
  Q_OUT_29 (1 BIT) : Inport  Port=30
  Q_OUT_30 (1 BIT) : Inport  Port=31
  Q_OUT_31 (1 BIT) : Inport  Port=32
  Concat{1,3,6,8..30} (26 alike) : hdlBasic/Concat  num_inputs=2  XmcBlockStatus=1  maskContainerNames=group1  block_type=concat  block_config=sysgen:Concat_config
  IN_00 : hdlBasic/Concat  num_inputs=2  XmcBlockStatus=1  maskContainerNames=group1  block_type=concat  block_config=sysgen:Concat_config
  IN_01 : hdlBasic/Concat  num_inputs=2  XmcBlockStatus=1  maskContainerNames=group1  block_type=concat  block_config=sysgen:Concat_config
  IN_02 : hdlBasic/Concat  num_inputs=2  XmcBlockStatus=1  maskContainerNames=group1  block_type=concat  block_config=sysgen:Concat_config
  IN_03 : hdlBasic/Concat  num_inputs=2  XmcBlockStatus=1  maskContainerNames=group1  block_type=concat  block_config=sysgen:Concat_config
  IN_04 : hdlBasic/Concat  num_inputs=2  XmcBlockStatus=1  maskContainerNames=group1  block_type=concat  block_config=sysgen:Concat_config
  Q (32 BIT) : Outport
  wires:
  IN_01/1 -> Concat3/2
  Concat10/1 -> Concat12/1
  Concat27/1 -> Concat20/2
  Concat19/1 -> Concat21/2
  Concat22/1 -> Concat1/2
  Concat28/1 -> Concat30/1
  Concat11/1 -> Concat12/2
  Concat29/1 -> Concat30/2
  Concat21/1 -> Concat22/2
  IN_00/1 -> Concat3/1
  Concat3/1 -> Concat13/1
  Concat20/1 -> Concat22/1
  Concat17/1 -> Concat19/1
  Concat26/1 -> Concat27/2
  Concat6/1 -> Concat13/2
  Concat13/1 -> Concat15/1
  Concat30/1 -> Concat21/1
  Concat24/1 -> Concat20/1
  Concat16/1 -> Concat24/1
  Concat23/1 -> Concat24/2
  Concat18/1 -> Concat19/2
  Concat25/1 -> Concat27/1
  IN_02/1 -> Concat6/1
  IN_03/1 -> Concat6/2
  Concat9/1 -> Concat14/1
  Concat15/1 -> Concat1/1
  Concat8/1 -> Concat9/2
  IN_04/1 -> Concat9/1
  Concat14/1 -> Concat15/2
  Concat12/1 -> Concat14/2
  Concat1/1 -> Q (32 BIT)/1
  Q_OUT_31 (1 BIT)/1 -> IN_00/1
  Q_OUT_30 (1 BIT)/1 -> IN_00/2
  Q_OUT_29 (1 BIT)/1 -> IN_01/1
  Q_OUT_28 (1 BIT)/1 -> IN_01/2
  Q_OUT_27 (1 BIT)/1 -> IN_02/1
  Q_OUT_26 (1 BIT)/1 -> IN_02/2
  Q_OUT_25 (1 BIT)/1 -> IN_03/1
  Q_OUT_24 (1 BIT)/1 -> IN_03/2
  Q_OUT_23 (1 BIT)/1 -> IN_04/1
  Q_OUT_22 (1 BIT)/1 -> IN_04/2
  Q_OUT_21 (1 BIT)/1 -> Concat8/1
  Q_OUT_20 (1 BIT)/1 -> Concat8/2
  Q_OUT_19 (1 BIT)/1 -> Concat10/1
  Q_OUT_18 (1 BIT)/1 -> Concat10/2
  Q_OUT_17 (1 BIT)/1 -> Concat11/1
  Q_OUT_16 (1 BIT)/1 -> Concat11/2
  Q_OUT_15 (1 BIT)/1 -> Concat16/1
  Q_OUT_14 (1 BIT)/1 -> Concat16/2
  Q_OUT_13 (1 BIT)/1 -> Concat23/1
  Q_OUT_12 (1 BIT)/1 -> Concat23/2
  Q_OUT_11 (1 BIT)/1 -> Concat25/1
  Q_OUT_10 (1 BIT)/1 -> Concat25/2
  Q_OUT_9 (1 BIT)/1 -> Concat26/1
  Q_OUT_8 (1 BIT)/1 -> Concat26/2
  Q_OUT_7 (1 BIT)/1 -> Concat28/1
  Q_OUT_6 (1 BIT)/1 -> Concat28/2
  Q_OUT_5 (1 BIT)/1 -> Concat29/1
  Q_OUT_4 (1 BIT)/1 -> Concat29/2
  Q_OUT_3 (1 BIT)/1 -> Concat17/1
  Q_OUT_2 (1 BIT)/1 -> Concat17/2
  Q_OUT_1 (1 BIT)/1 -> Concat18/1
  Q_OUT_0 (1 BIT)/1 -> Concat18/2

== system REGISTROS_64_BITS_02/REGISTRO_64_BITS_23/Q_OUT_32_BIT1 ==
  Q_OUT_0 (1 BIT) : Inport
  Q_OUT_1 (1 BIT) : Inport  Port=2
  Q_OUT_2 (1 BIT) : Inport  Port=3
  Q_OUT_3 (1 BIT) : Inport  Port=4
  Q_OUT_4 (1 BIT) : Inport  Port=5
  Q_OUT_5 (1 BIT) : Inport  Port=6
  Q_OUT_6 (1 BIT) : Inport  Port=7
  Q_OUT_7 (1 BIT) : Inport  Port=8
  Q_OUT_8 (1 BIT) : Inport  Port=9
  Q_OUT_9 (1 BIT) : Inport  Port=10
  Q_OUT_10 (1 BIT) : Inport  Port=11
  Q_OUT_11 (1 BIT) : Inport  Port=12
  Q_OUT_12 (1 BIT) : Inport  Port=13
  Q_OUT_13 (1 BIT) : Inport  Port=14
  Q_OUT_14 (1 BIT) : Inport  Port=15
  Q_OUT_15 (1 BIT) : Inport  Port=16
  Q_OUT_16 (1 BIT) : Inport  Port=17
  Q_OUT_17 (1 BIT) : Inport  Port=18
  Q_OUT_18 (1 BIT) : Inport  Port=19
  Q_OUT_19 (1 BIT) : Inport  Port=20
  Q_OUT_20 (1 BIT) : Inport  Port=21
  Q_OUT_21 (1 BIT) : Inport  Port=22
  Q_OUT_22 (1 BIT) : Inport  Port=23
  Q_OUT_23 (1 BIT) : Inport  Port=24
  Q_OUT_24 (1 BIT) : Inport  Port=25
  Q_OUT_25 (1 BIT) : Inport  Port=26
  Q_OUT_26 (1 BIT) : Inport  Port=27
  Q_OUT_27 (1 BIT) : Inport  Port=28
  Q_OUT_28 (1 BIT) : Inport  Port=29
  Q_OUT_29 (1 BIT) : Inport  Port=30
  Q_OUT_30 (1 BIT) : Inport  Port=31
  Q_OUT_31 (1 BIT) : Inport  Port=32
  Concat{1,3,6,8..30} (26 alike) : hdlBasic/Concat  num_inputs=2  XmcBlockStatus=1  maskContainerNames=group1  block_type=concat  block_config=sysgen:Concat_config
  IN_00 : hdlBasic/Concat  num_inputs=2  XmcBlockStatus=1  maskContainerNames=group1  block_type=concat  block_config=sysgen:Concat_config
  IN_01 : hdlBasic/Concat  num_inputs=2  XmcBlockStatus=1  maskContainerNames=group1  block_type=concat  block_config=sysgen:Concat_config
  IN_02 : hdlBasic/Concat  num_inputs=2  XmcBlockStatus=1  maskContainerNames=group1  block_type=concat  block_config=sysgen:Concat_config
  IN_03 : hdlBasic/Concat  num_inputs=2  XmcBlockStatus=1  maskContainerNames=group1  block_type=concat  block_config=sysgen:Concat_config
  IN_04 : hdlBasic/Concat  num_inputs=2  XmcBlockStatus=1  maskContainerNames=group1  block_type=concat  block_config=sysgen:Concat_config
  Q (32 BIT) : Outport
  wires:
  IN_01/1 -> Concat3/2
  Concat10/1 -> Concat12/1
  Concat27/1 -> Concat20/2
  Concat19/1 -> Concat21/2
  Concat22/1 -> Concat1/2
  Concat28/1 -> Concat30/1
  Concat11/1 -> Concat12/2
  Concat29/1 -> Concat30/2
  Concat21/1 -> Concat22/2
  IN_00/1 -> Concat3/1
  Concat3/1 -> Concat13/1
  Concat20/1 -> Concat22/1
  Concat17/1 -> Concat19/1
  Concat26/1 -> Concat27/2
  Concat6/1 -> Concat13/2
  Concat13/1 -> Concat15/1
  Concat30/1 -> Concat21/1
  Concat24/1 -> Concat20/1
  Concat16/1 -> Concat24/1
  Concat23/1 -> Concat24/2
  Concat18/1 -> Concat19/2
  Concat25/1 -> Concat27/1
  IN_02/1 -> Concat6/1
  IN_03/1 -> Concat6/2
  Concat9/1 -> Concat14/1
  Concat15/1 -> Concat1/1
  Concat8/1 -> Concat9/2
  IN_04/1 -> Concat9/1
  Concat14/1 -> Concat15/2
  Concat12/1 -> Concat14/2
  Concat1/1 -> Q (32 BIT)/1
  Q_OUT_31 (1 BIT)/1 -> IN_00/1
  Q_OUT_30 (1 BIT)/1 -> IN_00/2
  Q_OUT_29 (1 BIT)/1 -> IN_01/1
  Q_OUT_28 (1 BIT)/1 -> IN_01/2
  Q_OUT_27 (1 BIT)/1 -> IN_02/1
  Q_OUT_26 (1 BIT)/1 -> IN_02/2
  Q_OUT_25 (1 BIT)/1 -> IN_03/1
  Q_OUT_24 (1 BIT)/1 -> IN_03/2
  Q_OUT_23 (1 BIT)/1 -> IN_04/1
  Q_OUT_22 (1 BIT)/1 -> IN_04/2
  Q_OUT_21 (1 BIT)/1 -> Concat8/1
  Q_OUT_20 (1 BIT)/1 -> Concat8/2
  Q_OUT_19 (1 BIT)/1 -> Concat10/1
  Q_OUT_18 (1 BIT)/1 -> Concat10/2
  Q_OUT_17 (1 BIT)/1 -> Concat11/1
  Q_OUT_16 (1 BIT)/1 -> Concat11/2
  Q_OUT_15 (1 BIT)/1 -> Concat16/1
  Q_OUT_14 (1 BIT)/1 -> Concat16/2
  Q_OUT_13 (1 BIT)/1 -> Concat23/1
  Q_OUT_12 (1 BIT)/1 -> Concat23/2
  Q_OUT_11 (1 BIT)/1 -> Concat25/1
  Q_OUT_10 (1 BIT)/1 -> Concat25/2
  Q_OUT_9 (1 BIT)/1 -> Concat26/1
  Q_OUT_8 (1 BIT)/1 -> Concat26/2
  Q_OUT_7 (1 BIT)/1 -> Concat28/1
  Q_OUT_6 (1 BIT)/1 -> Concat28/2
  Q_OUT_5 (1 BIT)/1 -> Concat29/1
  Q_OUT_4 (1 BIT)/1 -> Concat29/2
  Q_OUT_3 (1 BIT)/1 -> Concat17/1
  Q_OUT_2 (1 BIT)/1 -> Concat17/2
  Q_OUT_1 (1 BIT)/1 -> Concat18/1
  Q_OUT_0 (1 BIT)/1 -> Concat18/2

== system REGISTROS_64_BITS_02/REGISTRO_64_BITS_23/Q_OUT_32_BIT2 ==
  Q_OUT_0 (1 BIT) : Inport
  Q_OUT_1 (1 BIT) : Inport  Port=2
  Q_OUT_2 (1 BIT) : Inport  Port=3
  Q_OUT_3 (1 BIT) : Inport  Port=4
  Q_OUT_4 (1 BIT) : Inport  Port=5
  Q_OUT_5 (1 BIT) : Inport  Port=6
  Q_OUT_6 (1 BIT) : Inport  Port=7
  Q_OUT_7 (1 BIT) : Inport  Port=8
  Q_OUT_8 (1 BIT) : Inport  Port=9
  Q_OUT_9 (1 BIT) : Inport  Port=10
  Q_OUT_10 (1 BIT) : Inport  Port=11
  Q_OUT_11 (1 BIT) : Inport  Port=12
  Q_OUT_12 (1 BIT) : Inport  Port=13
  Q_OUT_13 (1 BIT) : Inport  Port=14
  Q_OUT_14 (1 BIT) : Inport  Port=15
  Q_OUT_15 (1 BIT) : Inport  Port=16
  Q_OUT_16 (1 BIT) : Inport  Port=17
  Q_OUT_17 (1 BIT) : Inport  Port=18
  Q_OUT_18 (1 BIT) : Inport  Port=19
  Q_OUT_19 (1 BIT) : Inport  Port=20
  Q_OUT_20 (1 BIT) : Inport  Port=21
  Q_OUT_21 (1 BIT) : Inport  Port=22
  Q_OUT_22 (1 BIT) : Inport  Port=23
  Q_OUT_23 (1 BIT) : Inport  Port=24
  Q_OUT_24 (1 BIT) : Inport  Port=25
  Q_OUT_25 (1 BIT) : Inport  Port=26
  Q_OUT_26 (1 BIT) : Inport  Port=27
  Q_OUT_27 (1 BIT) : Inport  Port=28
  Q_OUT_28 (1 BIT) : Inport  Port=29
  Q_OUT_29 (1 BIT) : Inport  Port=30
  Q_OUT_30 (1 BIT) : Inport  Port=31
  Q_OUT_31 (1 BIT) : Inport  Port=32
  Concat{1,3,6,8..30} (26 alike) : hdlBasic/Concat  num_inputs=2  XmcBlockStatus=1  maskContainerNames=group1  block_type=concat  block_config=sysgen:Concat_config
  IN_00 : hdlBasic/Concat  num_inputs=2  XmcBlockStatus=1  maskContainerNames=group1  block_type=concat  block_config=sysgen:Concat_config
  IN_01 : hdlBasic/Concat  num_inputs=2  XmcBlockStatus=1  maskContainerNames=group1  block_type=concat  block_config=sysgen:Concat_config
  IN_02 : hdlBasic/Concat  num_inputs=2  XmcBlockStatus=1  maskContainerNames=group1  block_type=concat  block_config=sysgen:Concat_config
  IN_03 : hdlBasic/Concat  num_inputs=2  XmcBlockStatus=1  maskContainerNames=group1  block_type=concat  block_config=sysgen:Concat_config
  IN_04 : hdlBasic/Concat  num_inputs=2  XmcBlockStatus=1  maskContainerNames=group1  block_type=concat  block_config=sysgen:Concat_config
  Q (32 BIT) : Outport
  wires:
  IN_01/1 -> Concat3/2
  Concat10/1 -> Concat12/1
  Concat27/1 -> Concat20/2
  Concat19/1 -> Concat21/2
  Concat22/1 -> Concat1/2
  Concat28/1 -> Concat30/1
  Concat11/1 -> Concat12/2
  Concat29/1 -> Concat30/2
  Concat21/1 -> Concat22/2
  IN_00/1 -> Concat3/1
  Concat3/1 -> Concat13/1
  Concat20/1 -> Concat22/1
  Concat17/1 -> Concat19/1
  Concat26/1 -> Concat27/2
  Concat6/1 -> Concat13/2
  Concat13/1 -> Concat15/1
  Concat30/1 -> Concat21/1
  Concat24/1 -> Concat20/1
  Concat16/1 -> Concat24/1
  Concat23/1 -> Concat24/2
  Concat18/1 -> Concat19/2
  Concat25/1 -> Concat27/1
  IN_02/1 -> Concat6/1
  IN_03/1 -> Concat6/2
  Concat9/1 -> Concat14/1
  Concat15/1 -> Concat1/1
  Concat8/1 -> Concat9/2
  IN_04/1 -> Concat9/1
  Concat14/1 -> Concat15/2
  Concat12/1 -> Concat14/2
  Concat1/1 -> Q (32 BIT)/1
  Q_OUT_31 (1 BIT)/1 -> IN_00/1
  Q_OUT_30 (1 BIT)/1 -> IN_00/2
  Q_OUT_29 (1 BIT)/1 -> IN_01/1
  Q_OUT_28 (1 BIT)/1 -> IN_01/2
  Q_OUT_27 (1 BIT)/1 -> IN_02/1
  Q_OUT_26 (1 BIT)/1 -> IN_02/2
  Q_OUT_25 (1 BIT)/1 -> IN_03/1
  Q_OUT_24 (1 BIT)/1 -> IN_03/2
  Q_OUT_23 (1 BIT)/1 -> IN_04/1
  Q_OUT_22 (1 BIT)/1 -> IN_04/2
  Q_OUT_21 (1 BIT)/1 -> Concat8/1
  Q_OUT_20 (1 BIT)/1 -> Concat8/2
  Q_OUT_19 (1 BIT)/1 -> Concat10/1
  Q_OUT_18 (1 BIT)/1 -> Concat10/2
  Q_OUT_17 (1 BIT)/1 -> Concat11/1
  Q_OUT_16 (1 BIT)/1 -> Concat11/2
  Q_OUT_15 (1 BIT)/1 -> Concat16/1
  Q_OUT_14 (1 BIT)/1 -> Concat16/2
  Q_OUT_13 (1 BIT)/1 -> Concat23/1
  Q_OUT_12 (1 BIT)/1 -> Concat23/2
  Q_OUT_11 (1 BIT)/1 -> Concat25/1
  Q_OUT_10 (1 BIT)/1 -> Concat25/2
  Q_OUT_9 (1 BIT)/1 -> Concat26/1
  Q_OUT_8 (1 BIT)/1 -> Concat26/2
  Q_OUT_7 (1 BIT)/1 -> Concat28/1
  Q_OUT_6 (1 BIT)/1 -> Concat28/2
  Q_OUT_5 (1 BIT)/1 -> Concat29/1
  Q_OUT_4 (1 BIT)/1 -> Concat29/2
  Q_OUT_3 (1 BIT)/1 -> Concat17/1
  Q_OUT_2 (1 BIT)/1 -> Concat17/2
  Q_OUT_1 (1 BIT)/1 -> Concat18/1
  Q_OUT_0 (1 BIT)/1 -> Concat18/2

== system REGISTROS_64_BITS_02/REGISTRO_64_BITS_24/Q_OUT_32_BIT1 ==
  Q_OUT_0 (1 BIT) : Inport
  Q_OUT_1 (1 BIT) : Inport  Port=2
  Q_OUT_2 (1 BIT) : Inport  Port=3
  Q_OUT_3 (1 BIT) : Inport  Port=4
  Q_OUT_4 (1 BIT) : Inport  Port=5
  Q_OUT_5 (1 BIT) : Inport  Port=6
  Q_OUT_6 (1 BIT) : Inport  Port=7
  Q_OUT_7 (1 BIT) : Inport  Port=8
  Q_OUT_8 (1 BIT) : Inport  Port=9
  Q_OUT_9 (1 BIT) : Inport  Port=10
  Q_OUT_10 (1 BIT) : Inport  Port=11
  Q_OUT_11 (1 BIT) : Inport  Port=12
  Q_OUT_12 (1 BIT) : Inport  Port=13
  Q_OUT_13 (1 BIT) : Inport  Port=14
  Q_OUT_14 (1 BIT) : Inport  Port=15
  Q_OUT_15 (1 BIT) : Inport  Port=16
  Q_OUT_16 (1 BIT) : Inport  Port=17
  Q_OUT_17 (1 BIT) : Inport  Port=18
  Q_OUT_18 (1 BIT) : Inport  Port=19
  Q_OUT_19 (1 BIT) : Inport  Port=20
  Q_OUT_20 (1 BIT) : Inport  Port=21
  Q_OUT_21 (1 BIT) : Inport  Port=22
  Q_OUT_22 (1 BIT) : Inport  Port=23
  Q_OUT_23 (1 BIT) : Inport  Port=24
  Q_OUT_24 (1 BIT) : Inport  Port=25
  Q_OUT_25 (1 BIT) : Inport  Port=26
  Q_OUT_26 (1 BIT) : Inport  Port=27
  Q_OUT_27 (1 BIT) : Inport  Port=28
  Q_OUT_28 (1 BIT) : Inport  Port=29
  Q_OUT_29 (1 BIT) : Inport  Port=30
  Q_OUT_30 (1 BIT) : Inport  Port=31
  Q_OUT_31 (1 BIT) : Inport  Port=32
  Concat{1,3,6,8..30} (26 alike) : hdlBasic/Concat  num_inputs=2  XmcBlockStatus=1  maskContainerNames=group1  block_type=concat  block_config=sysgen:Concat_config
  IN_00 : hdlBasic/Concat  num_inputs=2  XmcBlockStatus=1  maskContainerNames=group1  block_type=concat  block_config=sysgen:Concat_config
  IN_01 : hdlBasic/Concat  num_inputs=2  XmcBlockStatus=1  maskContainerNames=group1  block_type=concat  block_config=sysgen:Concat_config
  IN_02 : hdlBasic/Concat  num_inputs=2  XmcBlockStatus=1  maskContainerNames=group1  block_type=concat  block_config=sysgen:Concat_config
  IN_03 : hdlBasic/Concat  num_inputs=2  XmcBlockStatus=1  maskContainerNames=group1  block_type=concat  block_config=sysgen:Concat_config
  IN_04 : hdlBasic/Concat  num_inputs=2  XmcBlockStatus=1  maskContainerNames=group1  block_type=concat  block_config=sysgen:Concat_config
  Q (32 BIT) : Outport
  wires:
  IN_01/1 -> Concat3/2
  Concat10/1 -> Concat12/1
  Concat27/1 -> Concat20/2
  Concat19/1 -> Concat21/2
  Concat22/1 -> Concat1/2
  Concat28/1 -> Concat30/1
  Concat11/1 -> Concat12/2
  Concat29/1 -> Concat30/2
  Concat21/1 -> Concat22/2
  IN_00/1 -> Concat3/1
  Concat3/1 -> Concat13/1
  Concat20/1 -> Concat22/1
  Concat17/1 -> Concat19/1
  Concat26/1 -> Concat27/2
  Concat6/1 -> Concat13/2
  Concat13/1 -> Concat15/1
  Concat30/1 -> Concat21/1
  Concat24/1 -> Concat20/1
  Concat16/1 -> Concat24/1
  Concat23/1 -> Concat24/2
  Concat18/1 -> Concat19/2
  Concat25/1 -> Concat27/1
  IN_02/1 -> Concat6/1
  IN_03/1 -> Concat6/2
  Concat9/1 -> Concat14/1
  Concat15/1 -> Concat1/1
  Concat8/1 -> Concat9/2
  IN_04/1 -> Concat9/1
  Concat14/1 -> Concat15/2
  Concat12/1 -> Concat14/2
  Concat1/1 -> Q (32 BIT)/1
  Q_OUT_31 (1 BIT)/1 -> IN_00/1
  Q_OUT_30 (1 BIT)/1 -> IN_00/2
  Q_OUT_29 (1 BIT)/1 -> IN_01/1
  Q_OUT_28 (1 BIT)/1 -> IN_01/2
  Q_OUT_27 (1 BIT)/1 -> IN_02/1
  Q_OUT_26 (1 BIT)/1 -> IN_02/2
  Q_OUT_25 (1 BIT)/1 -> IN_03/1
  Q_OUT_24 (1 BIT)/1 -> IN_03/2
  Q_OUT_23 (1 BIT)/1 -> IN_04/1
  Q_OUT_22 (1 BIT)/1 -> IN_04/2
  Q_OUT_21 (1 BIT)/1 -> Concat8/1
  Q_OUT_20 (1 BIT)/1 -> Concat8/2
  Q_OUT_19 (1 BIT)/1 -> Concat10/1
  Q_OUT_18 (1 BIT)/1 -> Concat10/2
  Q_OUT_17 (1 BIT)/1 -> Concat11/1
  Q_OUT_16 (1 BIT)/1 -> Concat11/2
  Q_OUT_15 (1 BIT)/1 -> Concat16/1
  Q_OUT_14 (1 BIT)/1 -> Concat16/2
  Q_OUT_13 (1 BIT)/1 -> Concat23/1
  Q_OUT_12 (1 BIT)/1 -> Concat23/2
  Q_OUT_11 (1 BIT)/1 -> Concat25/1
  Q_OUT_10 (1 BIT)/1 -> Concat25/2
  Q_OUT_9 (1 BIT)/1 -> Concat26/1
  Q_OUT_8 (1 BIT)/1 -> Concat26/2
  Q_OUT_7 (1 BIT)/1 -> Concat28/1
  Q_OUT_6 (1 BIT)/1 -> Concat28/2
  Q_OUT_5 (1 BIT)/1 -> Concat29/1
  Q_OUT_4 (1 BIT)/1 -> Concat29/2
  Q_OUT_3 (1 BIT)/1 -> Concat17/1
  Q_OUT_2 (1 BIT)/1 -> Concat17/2
  Q_OUT_1 (1 BIT)/1 -> Concat18/1
  Q_OUT_0 (1 BIT)/1 -> Concat18/2

== system REGISTROS_64_BITS_02/REGISTRO_64_BITS_24/Q_OUT_32_BIT2 ==
  Q_OUT_0 (1 BIT) : Inport
  Q_OUT_1 (1 BIT) : Inport  Port=2
  Q_OUT_2 (1 BIT) : Inport  Port=3
  Q_OUT_3 (1 BIT) : Inport  Port=4
  Q_OUT_4 (1 BIT) : Inport  Port=5
  Q_OUT_5 (1 BIT) : Inport  Port=6
  Q_OUT_6 (1 BIT) : Inport  Port=7
  Q_OUT_7 (1 BIT) : Inport  Port=8
  Q_OUT_8 (1 BIT) : Inport  Port=9
  Q_OUT_9 (1 BIT) : Inport  Port=10
  Q_OUT_10 (1 BIT) : Inport  Port=11
  Q_OUT_11 (1 BIT) : Inport  Port=12
  Q_OUT_12 (1 BIT) : Inport  Port=13
  Q_OUT_13 (1 BIT) : Inport  Port=14
  Q_OUT_14 (1 BIT) : Inport  Port=15
  Q_OUT_15 (1 BIT) : Inport  Port=16
  Q_OUT_16 (1 BIT) : Inport  Port=17
  Q_OUT_17 (1 BIT) : Inport  Port=18
  Q_OUT_18 (1 BIT) : Inport  Port=19
  Q_OUT_19 (1 BIT) : Inport  Port=20
  Q_OUT_20 (1 BIT) : Inport  Port=21
  Q_OUT_21 (1 BIT) : Inport  Port=22
  Q_OUT_22 (1 BIT) : Inport  Port=23
  Q_OUT_23 (1 BIT) : Inport  Port=24
  Q_OUT_24 (1 BIT) : Inport  Port=25
  Q_OUT_25 (1 BIT) : Inport  Port=26
  Q_OUT_26 (1 BIT) : Inport  Port=27
  Q_OUT_27 (1 BIT) : Inport  Port=28
  Q_OUT_28 (1 BIT) : Inport  Port=29
  Q_OUT_29 (1 BIT) : Inport  Port=30
  Q_OUT_30 (1 BIT) : Inport  Port=31
  Q_OUT_31 (1 BIT) : Inport  Port=32
  Concat{1,3,6,8..30} (26 alike) : hdlBasic/Concat  num_inputs=2  XmcBlockStatus=1  maskContainerNames=group1  block_type=concat  block_config=sysgen:Concat_config
  IN_00 : hdlBasic/Concat  num_inputs=2  XmcBlockStatus=1  maskContainerNames=group1  block_type=concat  block_config=sysgen:Concat_config
  IN_01 : hdlBasic/Concat  num_inputs=2  XmcBlockStatus=1  maskContainerNames=group1  block_type=concat  block_config=sysgen:Concat_config
  IN_02 : hdlBasic/Concat  num_inputs=2  XmcBlockStatus=1  maskContainerNames=group1  block_type=concat  block_config=sysgen:Concat_config
  IN_03 : hdlBasic/Concat  num_inputs=2  XmcBlockStatus=1  maskContainerNames=group1  block_type=concat  block_config=sysgen:Concat_config
  IN_04 : hdlBasic/Concat  num_inputs=2  XmcBlockStatus=1  maskContainerNames=group1  block_type=concat  block_config=sysgen:Concat_config
  Q (32 BIT) : Outport
  wires:
  IN_01/1 -> Concat3/2
  Concat10/1 -> Concat12/1
  Concat27/1 -> Concat20/2
  Concat19/1 -> Concat21/2
  Concat22/1 -> Concat1/2
  Concat28/1 -> Concat30/1
  Concat11/1 -> Concat12/2
  Concat29/1 -> Concat30/2
  Concat21/1 -> Concat22/2
  IN_00/1 -> Concat3/1
  Concat3/1 -> Concat13/1
  Concat20/1 -> Concat22/1
  Concat17/1 -> Concat19/1
  Concat26/1 -> Concat27/2
  Concat6/1 -> Concat13/2
  Concat13/1 -> Concat15/1
  Concat30/1 -> Concat21/1
  Concat24/1 -> Concat20/1
  Concat16/1 -> Concat24/1
  Concat23/1 -> Concat24/2
  Concat18/1 -> Concat19/2
  Concat25/1 -> Concat27/1
  IN_02/1 -> Concat6/1
  IN_03/1 -> Concat6/2
  Concat9/1 -> Concat14/1
  Concat15/1 -> Concat1/1
  Concat8/1 -> Concat9/2
  IN_04/1 -> Concat9/1
  Concat14/1 -> Concat15/2
  Concat12/1 -> Concat14/2
  Concat1/1 -> Q (32 BIT)/1
  Q_OUT_31 (1 BIT)/1 -> IN_00/1
  Q_OUT_30 (1 BIT)/1 -> IN_00/2
  Q_OUT_29 (1 BIT)/1 -> IN_01/1
  Q_OUT_28 (1 BIT)/1 -> IN_01/2
  Q_OUT_27 (1 BIT)/1 -> IN_02/1
  Q_OUT_26 (1 BIT)/1 -> IN_02/2
  Q_OUT_25 (1 BIT)/1 -> IN_03/1
  Q_OUT_24 (1 BIT)/1 -> IN_03/2
  Q_OUT_23 (1 BIT)/1 -> IN_04/1
  Q_OUT_22 (1 BIT)/1 -> IN_04/2
  Q_OUT_21 (1 BIT)/1 -> Concat8/1
  Q_OUT_20 (1 BIT)/1 -> Concat8/2
  Q_OUT_19 (1 BIT)/1 -> Concat10/1
  Q_OUT_18 (1 BIT)/1 -> Concat10/2
  Q_OUT_17 (1 BIT)/1 -> Concat11/1
  Q_OUT_16 (1 BIT)/1 -> Concat11/2
  Q_OUT_15 (1 BIT)/1 -> Concat16/1
  Q_OUT_14 (1 BIT)/1 -> Concat16/2
  Q_OUT_13 (1 BIT)/1 -> Concat23/1
  Q_OUT_12 (1 BIT)/1 -> Concat23/2
  Q_OUT_11 (1 BIT)/1 -> Concat25/1
  Q_OUT_10 (1 BIT)/1 -> Concat25/2
  Q_OUT_9 (1 BIT)/1 -> Concat26/1
  Q_OUT_8 (1 BIT)/1 -> Concat26/2
  Q_OUT_7 (1 BIT)/1 -> Concat28/1
  Q_OUT_6 (1 BIT)/1 -> Concat28/2
  Q_OUT_5 (1 BIT)/1 -> Concat29/1
  Q_OUT_4 (1 BIT)/1 -> Concat29/2
  Q_OUT_3 (1 BIT)/1 -> Concat17/1
  Q_OUT_2 (1 BIT)/1 -> Concat17/2
  Q_OUT_1 (1 BIT)/1 -> Concat18/1
  Q_OUT_0 (1 BIT)/1 -> Concat18/2
